simulink model "kalmanfilter_total"  (R2024b)
settings: Solver=FixedStepAuto  StartTime=0.0  StopTime=10.0  FixedStep=1  RelTol=1e-3
undefined symbols (not defined in the file): A, B, C, D, I_a, Vk, Wk
settings Model: Creator=54238  LastModifiedBy=54238

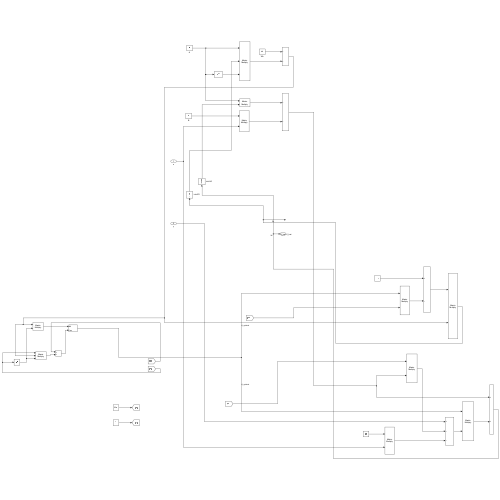
[thumbnail: Simulink's stored preview of the top-level diagram]
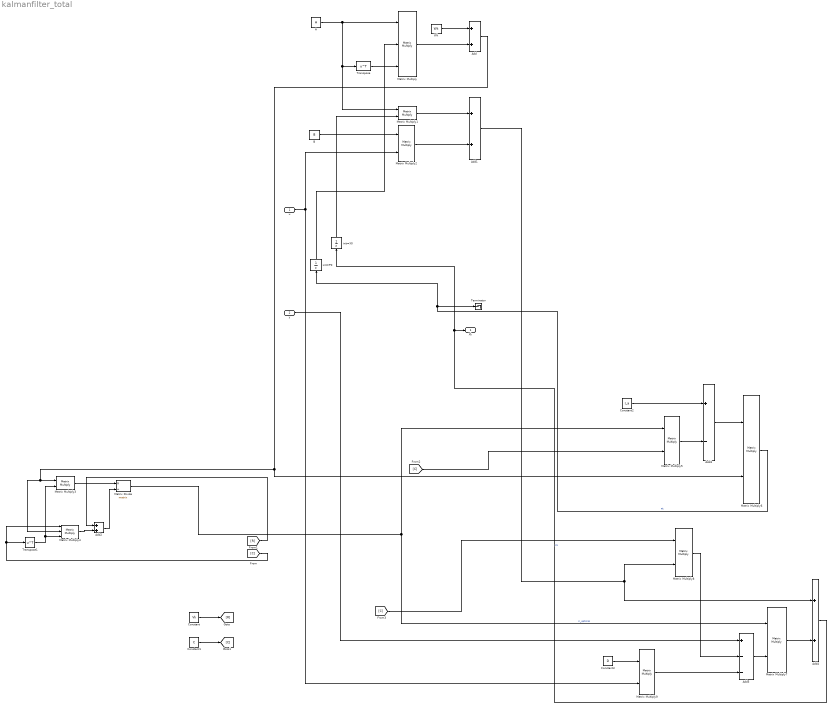
== system kalmanfilter_total ==
  u : Inport  PortDimensions=[2,1]
  y : Inport  Port=2  PortDimensions=[2,1]
  A : Constant  Value=A
  Add{,1..2,4} (4 alike) : Sum
  Add3 : Sum  Inputs=+-
  Add5 : Sum  Inputs=+--
  B : Constant  Value=B
  Constant : Constant  Value=Vk
  Constant1 : Constant  Value=C
  Constant2 : Constant  Value=I_a
  Constant3 : Constant  Value=D
  Matrix Divide : Product  Inputs=*/  Multiplication=Matrix(*)
  Matrix Multiply : Product  Inputs=3  Multiplication=Matrix(*)
  Matrix Multiply{1..3,5..9} (8 alike) : Product  Multiplication=Matrix(*)
  Matrix Multiply4 : Product  Inputs=3  Multiplication=Matrix(*)
  Terminator : Terminator
  Transpose : Math  Operator=transpose  SignedPower=on  RndMeth=Zero
  Transpose1 : Math  Operator=transpose
  Wk : Constant  Value=Wk
  init=P0 : UnitDelay  SampleTime=-1  StateName=p0  HasFrameUpgradeWarning=on
  init=X0 : UnitDelay  SampleTime=-1  HasFrameUpgradeWarning=on
  Xk : Outport  SignalName=X_hat  PortDimensions=[4,1]
  wires:
  Matrix Multiply6/1 -> init=P0/1, Terminator/1  "Pk"
  Add4/1 -> Xk/1, init=X0/1  "Xk"
  Transpose/1 -> Matrix Multiply/3
  init=P0/1 -> Matrix Multiply/2
  init=X0/1 -> Matrix Multiply1/2
  A/1 -> Matrix Multiply1/1, Transpose/1, Matrix Multiply/1
  Wk/1 -> Add/1
  Matrix Multiply2/1 -> Add1/2
  B/1 -> Matrix Multiply2/1
  Matrix Multiply/1 -> Add/2
  Matrix Multiply1/1 -> Add1/1
  Constant/1 -> [R]
  Constant1/1 -> [C]
  Matrix Divide/1 -> Matrix Multiply7/1, Matrix Multiply5/1  "K_optimal"
  [C] -> Matrix Multiply4/1, Transpose1/1
  Transpose1/1 -> Matrix Multiply4/3, Matrix Multiply3/2
  Matrix Multiply4/1 -> Add2/2
  Add2/1 -> Matrix Divide/2
  Matrix Multiply3/1 -> Matrix Divide/1
  [R] -> Add2/1
  Constant2/1 -> Add3/1
  Matrix Multiply5/1 -> Add3/2
  [C] -> Matrix Multiply5/2
  Add3/1 -> Matrix Multiply6/1
  Add/1 -> Matrix Multiply6/2, Matrix Multiply4/2, Matrix Multiply3/1
  u/1 -> Matrix Multiply9/2, Matrix Multiply2/2
  Add5/1 -> Matrix Multiply7/2
  y/1 -> Add5/1
  Add1/1 -> Matrix Multiply8/2, Add4/1
  Matrix Multiply9/1 -> Add5/3
  Matrix Multiply8/1 -> Add5/2
  Constant3/1 -> Matrix Multiply9/1
  [C] -> Matrix Multiply8/1
  Matrix Multiply7/1 -> Add4/2
